simulink model "getxy"  (Simulink 7.7)
settings: Solver=ode45  StartTime=0.0  StopTime=10.0  RelTol=1e-3
settings Model: Creator=Rachna  LastModifiedBy=Rachna

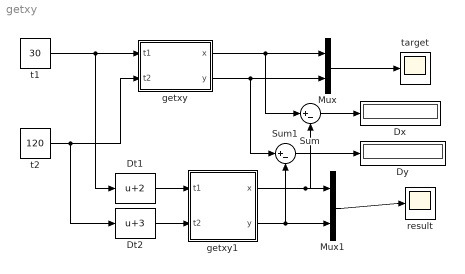
== system getxy ==
  Dt1 : Bias  Bias=2
  Dt2 : Bias  Bias=3
  Dx : Display
  Dy : Display
  Mux : Mux  Inputs=2
  Mux1 : Mux  Inputs=2
  Sum : Sum  Inputs=|+-
  Sum1 : Sum  Inputs=|+-
  getxy : Stateflow chart  TreatAsAtomicUnit=on
  getxy1 : Stateflow chart  TreatAsAtomicUnit=on
  result : Scope
  t1 : Constant  Value=30
  t2 : Constant  Value=120
  target : Scope
  wires:
  getxy/1(x) -> Sum/1, Mux/1
  getxy/2(y) -> Sum1/1, Mux/2
  t1/1 -> getxy/1(t1), Dt1/1
  t2/1 -> getxy/2(t2), Dt2/1
  Dt1/1 -> getxy1/1(t1)
  Dt2/1 -> getxy1/2(t2)
  getxy1/1(x) -> Sum/2, Mux1/1
  getxy1/2(y) -> Sum1/2, Mux1/2
  Mux1/1 -> result/1
  Sum/1 -> Dx/1
  Sum1/1 -> Dy/1
  Mux/1 -> target/1

== matlab function getxy ==
  data: x output double; t1 input double; y output double; t2 input double
function [ x, y ] = inverse(t1, t2)
%#codegen
t1 = (t1*pi)/180; %base angle
t2 = (t2*pi)/180; %elbow angle 
l1 = 30 ;         %upper arm length
l2 = 20 ;         %lower arm length
r = sqrt(l1*l1 + l2*l2 - cos(t2)*2*l1*l2) ; % distance between tip of arm and base
t0 = t1 - asin((l2*sin(t2))/r) ;      % angle of r with x axis
x = r*cos(t0);
y = r*sin(t0);

== matlab function getxy1 ==
  data: x output double; t1 input double; y output double; t2 input double
function [ x, y ] = inverse(t1, t2)
%#codegen
t1 = (t1*pi)/180; %base angle
t2 = (t2*pi)/180; %elbow angle 
l1 = 30 ;         %upper arm length
l2 = 20 ;         %lower arm length
r = sqrt(l1*l1 + l2*l2 - cos(t2)*2*l1*l2) ; % distance between tip of arm and base
t0 = t1 - asin((l2*sin(t2))/r) ;      % angle of r with x axis
x = r*cos(t0);
y = r*sin(t0);
